simulink model "Lab4a"  (R2019b)
settings: Solver=VariableStepAuto  StartTime=0.0  StopTime=10  RelTol=1e-3
libraries: commsynccomp2 x1, dspfdesign x1
settings Model: Creator=z3454314  LastModifiedBy=z3454314

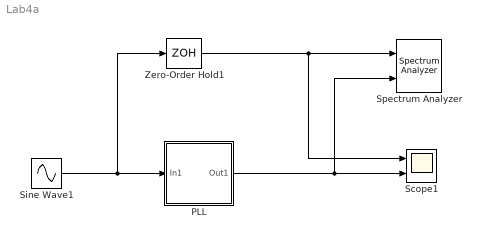
== system Lab4a ==
  "PLL " : Subsystem
  Scope1 : Scope  NumInputPorts=2
  Sine Wave1 : Sin  Frequency=8100*2*pi  SampleTime=0
  Spectrum Analyzer : SpectrumAnalyzer  NumInputPorts=2
  Zero-Order Hold1 : ZeroOrderHold  SampleTime=1/500e3
  wires:
  Zero-Order Hold1/1 -> Spectrum Analyzer/1, Scope1/1
  Sine Wave1/1 -> "PLL "/1(In1), Zero-Order Hold1/1
  "PLL "/1(Out1) -> Scope1/2, Spectrum Analyzer/2

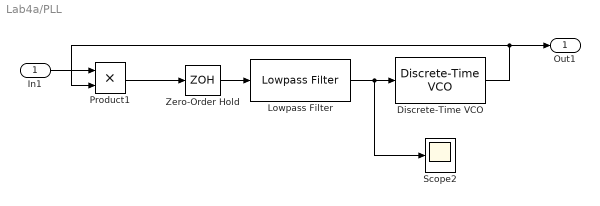
== system Lab4a/PLL  ==
  In1 : Inport
  Discrete-Time VCO : commsynccomp2/Discrete-Time VCO  Ac=1  Fc=8000  Kc=400  Ph=0  ts=1/500e3
      settings: SourceProductName=Communications Toolbox  SourceProductBaseCode=CM
  Lowpass Filter : dspfdesign/Lowpass Filter  FilterType=FIR  DesignForMinimumOrder=on  FilterOrder=50  PassbandFrequency=5e3  StopbandFrequency=10e3  PassbandRipple=0.1  StopbandAttenuation=80  InheritSampleRate=on  SampleRate=500e3  SimulateUsing=Interpreted execution  roundingMode=Floor  coeffsDataTypeStr=fixdt(1,16)
  Product1 : Product
  Scope2 : Scope
  Zero-Order Hold : ZeroOrderHold  SampleTime=1/500e3
  Out1 : Outport
  wires:
  Discrete-Time VCO/1 -> Out1/1, Product1/2
  Product1/1 -> Zero-Order Hold/1
  In1/1 -> Product1/1
  Lowpass Filter/1 -> Scope2/1, Discrete-Time VCO/1
  Zero-Order Hold/1 -> Lowpass Filter/1
